simulink model "cpusimuilater"  (R2020b)
settings: Solver=VariableStepAuto  StartTime=0.0  StopTime=inf  RelTol=1e-3
libraries: dspsigops x7
settings Model: Creator=nahomnegash  LastModifiedBy=nahomnegash

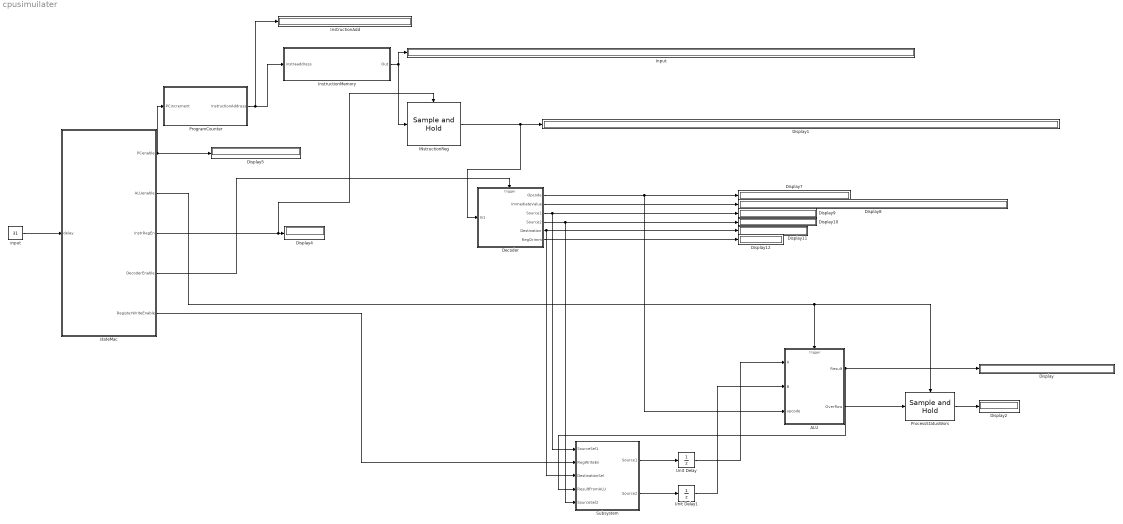
== system cpusimuilater ==
  ALU : Subsystem
  Decoder : Subsystem
  Display{,1..2,4..5,7..12} (11 alike) : Display
  INstructionReg : dspsigops/Sample and Hold  trig=Rising edge  initCond=0  latchinput=off
  Input : Display
  InstructionAdd : Display
  InstructionMemory : Subsystem
  ProcessStatusWors : dspsigops/Sample and Hold  trig=Rising edge  initCond=0  latchinput=off
  ProgramCounter : Subsystem
  Subsystem : Subsystem
  Unit Delay : UnitDelay  SampleTime=-1  HasFrameUpgradeWarning=on
  Unit Delay1 : UnitDelay  SampleTime=-1  HasFrameUpgradeWarning=on
  input : Constant  Value=31
  stateMac : Stateflow chart  TreatAsAtomicUnit=on
      settings: PortSchema="{\"entries\":[{\"content\":{\"sides\":[{\"content\":{\"connectorIds\":[\"In1\"]},\"type\":\"ConnectorPlacement.EquallySpacedRectSide\",\"uuid\":\"cf5c0f17-ae05-41cb-bb8a-264dbf8341ef\"},{\"content\":{\"connectorIds\":[\"Out1\",\"Out4\",\"Out2\",\"Out3\",\"Out5\"],\"side\":\"RIGHT\"},\"type\":\"ConnectorPlacement.EquallySpacedRectSide\",\"uuid\":\"f93a21af-1352-4f9d-82fe-283fa2f49b54\"},{\"content\":{\"connectorIds\":[],\"side\":\"TOP\"},\"type\":\"ConnectorPlacement.EquallySpacedRectSide\",\"uuid\":\"563b2710-7bdc-4fe1-815e-effac7f81df2\"}]},\"type\":\"ConnectorPlacement.EquallySpacedConnector\",\"uuid\":\"4ff43e67-6467-4fb9-af4e-bcbc08840be8\"}],\"packageUris\":[\"http://schema.mathworks.com/mf0/Connector/19700101\"],\"version\":\"1.0\"}"
  wires:
  ALU/1(Result) -> Subsystem/4(ResultFromALU), Display/1
  input/1 -> stateMac/1(delay)
  stateMac/2(InstrRegEn) -> INstructionReg/Trigger, Display4/1
  stateMac/3(DecoderEnable) -> Decoder/Trigger
  stateMac/4(ALUenable) -> ProcessStatusWors/Trigger, ALU/Trigger
  Decoder/2(ImmediateValue) -> Display8/1
  Decoder/3(Source1) -> Subsystem/1(SourceSel1), Display9/1
  Decoder/4(Source2) -> Subsystem/5(SourceSel2), Display10/1
  Decoder/5(Destination) -> Subsystem/3(DestinationSel), Display11/1
  Decoder/6(RegOrimm) -> Display12/1
  Decoder/1(Opcode) -> Display7/1, ALU/3(opcode)
  ALU/2(Overflow) -> ProcessStatusWors/1
  ProcessStatusWors/1 -> Display2/1
  InstructionMemory/1(Out) -> INstructionReg/1, Input/1
  stateMac/5(RegisterWriteEnable) -> Subsystem/2(RegWriteEn)
  INstructionReg/1 -> Decoder/1(In1), Display1/1
  stateMac/1(PCenable) -> Display5/1, ProgramCounter/1(PCincrement)
  ProgramCounter/1(InstructionAddress) -> InstructionMemory/1(instraaddress), InstructionAdd/1
  Subsystem/1(Source1) -> Unit Delay/1
  Unit Delay/1 -> ALU/1(A)
  Unit Delay1/1 -> ALU/2(B)
  Subsystem/2(Source2) -> Unit Delay1/1

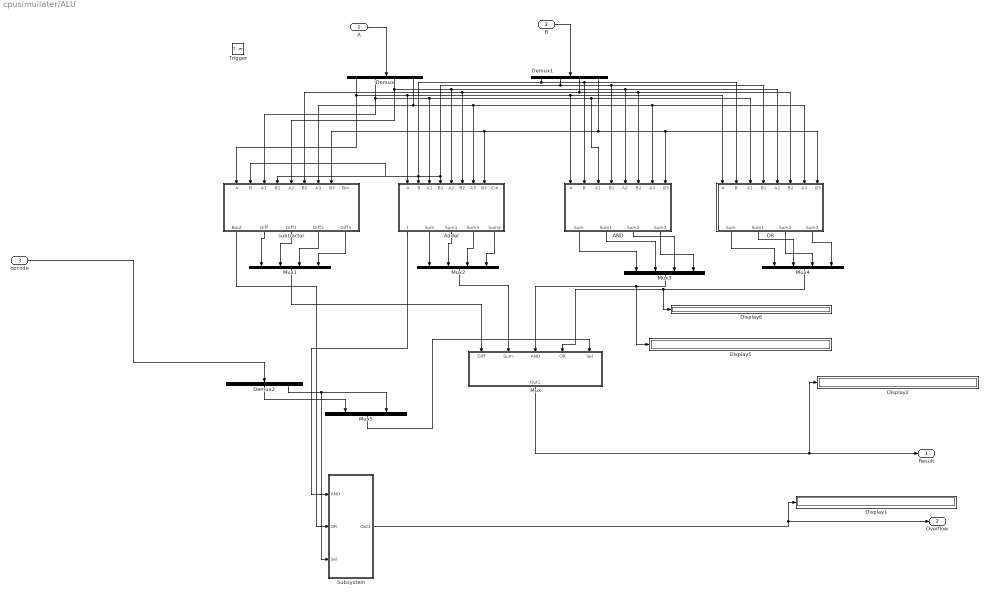
== system cpusimuilater/ALU ==
  A : Inport
  B : Inport  Port=2
  opcode : Inport  Port=3
  Trigger : TriggerPort  VariantControl=Variant  PortDimensions=1
  AND : Subsystem
  Adder : Subsystem
  Demux : Demux
  Demux1 : Demux
  Demux2 : Demux  Outputs=3
  Display{1..2,5..6} (4 alike) : Display
  Mux : Subsystem
  Mux{1..4} (4 alike) : Mux
  Mux5 : Mux  Inputs=2
  OR : Subsystem
  Subsystem : Subsystem
  subtractor : Subsystem
  Result : Outport
  Overflow : Outport  Port=2
  wires:
  A/1 -> Demux/1
  Mux2/1 -> Mux/2(Sum)
  AND/2(Sum1) -> Mux3/2
  Mux/1(Out1) -> Display2/1, Result/1
  Adder/1(CarryOut) -> Subsystem/1(AND)
  opcode/1 -> Demux2/1
  OR/4(Sum3) -> Mux4/4
  B/1 -> Demux1/1
  subtractor/1(Bout) -> Subsystem/2(OR)
  OR/1(Sum) -> Mux4/1
  Mux5/1 -> Mux/5(Sel)
  subtractor/5(Diff3) -> Mux1/4
  Mux4/1 -> Display6/1, Mux/4(OR)
  Mux3/1 -> Display5/1, Mux/3(AND)
  Adder/3(Sum1) -> Mux2/2
  Demux2/2 -> Mux5/1
  Adder/2(Sum) -> Mux2/1
  subtractor/2(Diff) -> Mux1/1
  Demux2/3 -> Subsystem/3(Sel), Mux5/2
  AND/1(Sum) -> Mux3/1
  Adder/5(Sum2) -> Mux2/4
  Mux1/1 -> Mux/1(Diff)
  OR/2(Sum1) -> Mux4/2
  AND/4(Sum3) -> Mux3/4
  subtractor/3(Diff1) -> Mux1/2
  OR/3(Sum2) -> Mux4/3
  subtractor/4(Diff2) -> Mux1/3
  AND/3(Sum2) -> Mux3/3
  Subsystem/1(Out1) -> Display1/1, Overflow/1
  Adder/4(Sum3) -> Mux2/3
  Demux1/4 -> subtractor/8(B3), Adder/8(B3), OR/8(B3), AND/8(B3)
  Demux/4 -> subtractor/7(A3), Adder/7(A3), AND/7(A3), OR/7(A3)
  Demux1/3 -> subtractor/6(B2), Adder/6(B2), AND/6(B2), OR/6(B2)
  Demux1/2 -> subtractor/4(B1), Adder/4(B1), AND/4(B1), OR/4(B1)
  Demux1/1 -> subtractor/2(B), Adder/2(B), AND/2(B), OR/2(B)
  Demux/3 -> subtractor/5(A2), Adder/5(A2), AND/5(A2), OR/5(A2)
  Demux/2 -> subtractor/3(A1), Adder/3(A1), OR/3(A1), AND/3(A1)
  Demux/1 -> subtractor/1(A), Adder/1(A), AND/1(A), OR/1(A)

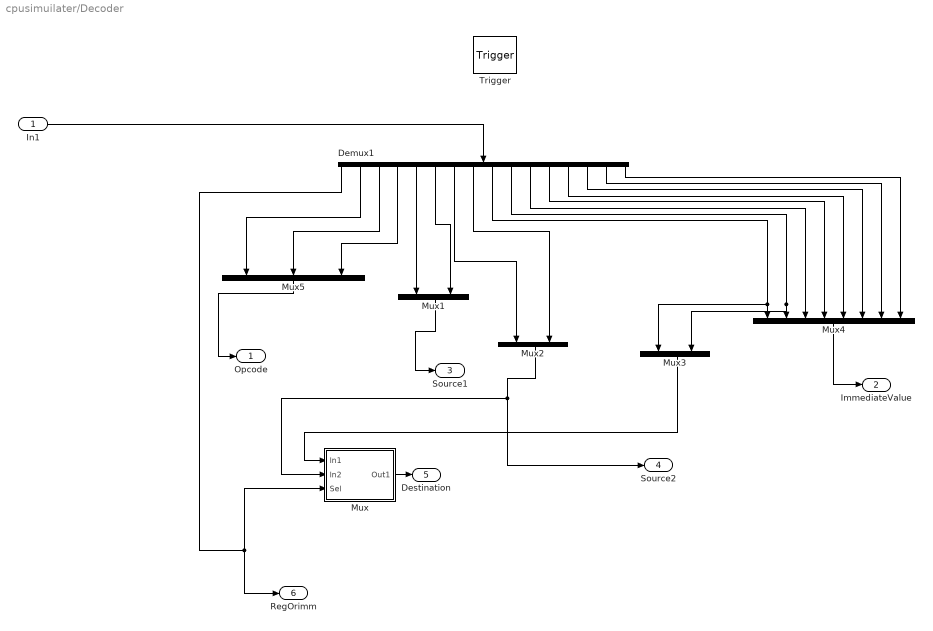
== system cpusimuilater/Decoder ==
  In1 : Inport
  Trigger : TriggerPort  VariantControl=Variant  PortDimensions=1
  Demux1 : Demux  Outputs=16
  Mux : Subsystem
  Mux1 : Mux  Inputs=2
  Mux2 : Mux  Inputs=2
  Mux3 : Mux  Inputs=2
  Mux4 : Mux  Inputs=8
  Mux5 : Mux  Inputs=3
  Opcode : Outport
  ImmediateValue : Outport  Port=2
  Source1 : Outport  Port=3
  Source2 : Outport  Port=4
  Destination : Outport  Port=5
  RegOrimm : Outport  Port=6
  wires:
  Demux1/13 -> Mux4/5
  Demux1/16 -> Mux4/8
  Mux3/1 -> Mux/1(ln1)
  Mux1/1 -> Source1/1
  Demux1/14 -> Mux4/6
  Demux1/6 -> Mux1/2
  Demux1/11 -> Mux4/3
  Demux1/7 -> Mux2/1
  In1/1 -> Demux1/1
  Demux1/9 -> Mux3/1, Mux4/1
  Demux1/4 -> Mux5/3
  Demux1/8 -> Mux2/2
  Demux1/3 -> Mux5/2
  Mux5/1 -> Opcode/1
  Demux1/10 -> Mux3/2, Mux4/2
  Mux2/1 -> Source2/1, Mux/2(ln2)
  Demux1/5 -> Mux1/1
  Mux/1(Out1) -> Destination/1
  Demux1/15 -> Mux4/7
  Demux1/1 -> RegOrimm/1, Mux/3(Sel)
  Mux4/1 -> ImmediateValue/1
  Demux1/12 -> Mux4/4
  Demux1/2 -> Mux5/1

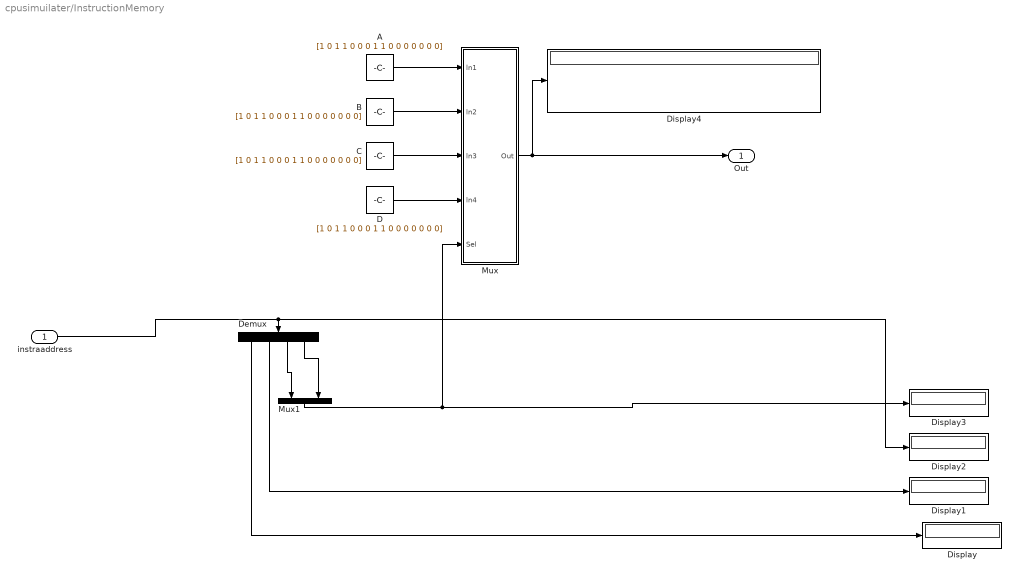
== system cpusimuilater/InstructionMemory ==
  instraaddress : Inport
  A : Constant  Value=[1 0 1 1 0 0 0 1 1 0 0 0 0 0 0 0]
  B : Constant  Value=[1 0 1 1 0 0 0 1 1 0 0 0 0 0 0 0]
  C : Constant  Value=[1 0 1 1 0 0 0 1 1 0 0 0 0 0 0 0]
  D : Constant  Value=[1 0 1 1 0 0 0 1 1 0 0 0 0 0 0 0]
  Demux : Demux
  Display{,1..4} (5 alike) : Display
  Mux : Subsystem
  Mux1 : Mux  Inputs=2
  Out : Outport
  wires:
  instraaddress/1 -> Display2/1, Demux/1
  Mux/1(Out) -> Out/1, Display4/1
  Demux/4 -> Mux1/2
  Demux/3 -> Mux1/1
  Mux1/1 -> Display3/1, Mux/5(Sel)
  A/1 -> Mux/1(ln1)
  B/1 -> Mux/2(ln2)
  C/1 -> Mux/3(ln3)
  D/1 -> Mux/4(ln4)
  Demux/1 -> Display/1
  Demux/2 -> Display1/1

== system cpusimuilater/ProgramCounter ==
  PCincrement : Inport
  Adder1 : Subsystem
  Constant : Constant
  Constant1 : Constant
  Demux : Demux
  Display : Display
  Display1 : Display
  Mux2 : Mux
  Sample and Hold : dspsigops/Sample and Hold  trig=Rising edge  initCond=0  latchinput=off
  Unit Delay : UnitDelay  SampleTime=-1  HasFrameUpgradeWarning=on
  InstructionAddress : Outport
  wires:
  Mux2/1 -> InstructionAddress/1, Display1/1, Unit Delay/1
  Adder1/1(CarryOut) -> Display/1
  Adder1/3(Sum1) -> Mux2/2
  Unit Delay/1 -> Sample and Hold/1
  Sample and Hold/1 -> Demux/1
  Adder1/2(Sum) -> Mux2/1
  Constant1/1 -> Adder1/9(C), Adder1/6(B2), Adder1/4(B1), Adder1/2(B)
  Adder1/5(Sum3) -> Mux2/4
  Demux/2 -> Adder1/3(A1)
  Adder1/4(Sum2) -> Mux2/3
  Constant/1 -> Adder1/8(B3)
  Demux/1 -> Adder1/1(A)
  Demux/3 -> Adder1/5(A2)
  Demux/4 -> Adder1/7(A3)
  PCincrement/1 -> Sample and Hold/Trigger

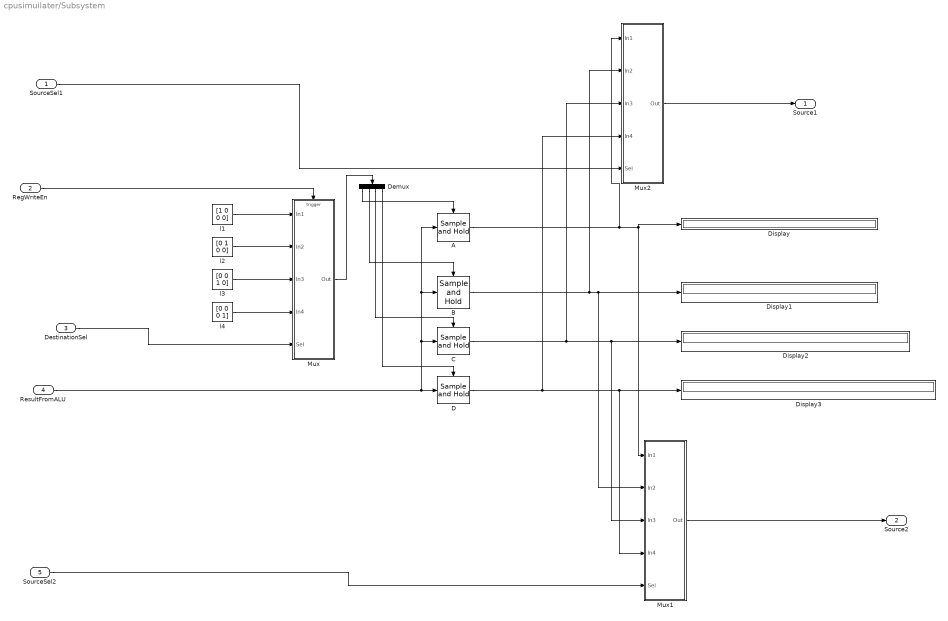
== system cpusimuilater/Subsystem ==
  SourceSel1 : Inport
  RegWriteEn : Inport  Port=2
  DestinationSel : Inport  Port=3
  ResultFromALU : Inport  Port=4
  SourceSel2 : Inport  Port=5
  A : dspsigops/Sample and Hold  trig=Rising edge  initCond=[1 0 0 0]  latchinput=off
  B : dspsigops/Sample and Hold  trig=Rising edge  initCond=[0 1 0 0]  latchinput=off
  C : dspsigops/Sample and Hold  trig=Rising edge  initCond=[0 0 1 0]  latchinput=off
  D : dspsigops/Sample and Hold  trig=Rising edge  initCond=[0 0 0 0]  latchinput=off
  Demux : Demux
  Display{,1..3} (4 alike) : Display
  Mux : Subsystem
  Mux1 : Subsystem
  Mux2 : Subsystem
  l1 : Constant  Value=[1 0 0 0]
  l2 : Constant  Value=[0 1 0 0]
  l3 : Constant  Value=[0 0 1 0]
  l4 : Constant  Value=[0 0 0 1]
  Source1 : Outport
  Source2 : Outport  Port=2
  wires:
  SourceSel1/1 -> Mux2/5(Sel)
  DestinationSel/1 -> Mux/5(Sel)
  Demux/4 -> D/Trigger
  l3/1 -> Mux/3(ln3)
  l2/1 -> Mux/2(ln2)
  Demux/3 -> C/Trigger
  Mux/1(Out) -> Demux/1
  l1/1 -> Mux/1(ln1)
  SourceSel2/1 -> Mux1/5(Sel)
  Mux1/1(Out) -> Source2/1
  l4/1 -> Mux/4(ln4)
  Demux/2 -> B/Trigger
  B/1 -> Display1/1, Mux1/2(ln2), Mux2/2(ln2)
  RegWriteEn/1 -> Mux/Trigger
  Mux2/1(Out) -> Source1/1
  D/1 -> Display3/1, Mux1/4(ln4), Mux2/4(ln4)
  A/1 -> Mux2/1(ln1), Mux1/1(ln1), Display/1
  Demux/1 -> A/Trigger
  ResultFromALU/1 -> A/1, B/1, C/1, D/1
  C/1 -> Display2/1, Mux1/3(ln3), Mux2/3(ln3)

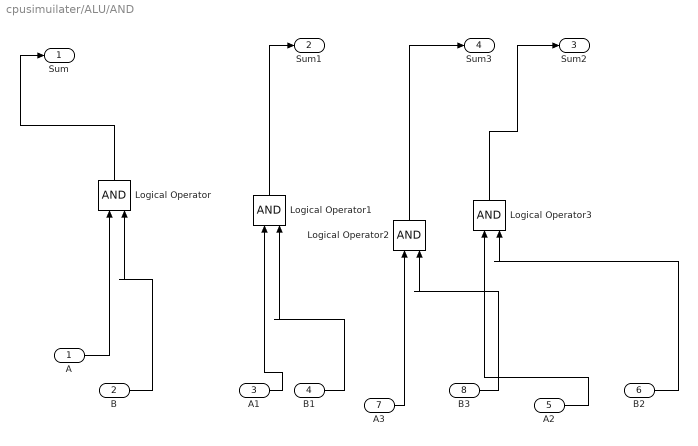
== system cpusimuilater/ALU/AND ==
  A : Inport
  B : Inport  Port=2
  A1 : Inport  Port=3
  B1 : Inport  Port=4
  A2 : Inport  Port=5
  B2 : Inport  Port=6
  A3 : Inport  Port=7
  B3 : Inport  Port=8
  Logical Operator{,1..3} (4 alike) : Logic  IconShape=distinctive  AllPortsSameDT=off  OutDataTypeStr=boolean
  Sum : Outport
  Sum1 : Outport  Port=2
  Sum2 : Outport  Port=3
  Sum3 : Outport  Port=4
  wires:
  A2/1 -> Logical Operator3/1
  Logical Operator2/1 -> Sum3/1
  B/1 -> Logical Operator/2
  B1/1 -> Logical Operator1/2
  A1/1 -> Logical Operator1/1
  B2/1 -> Logical Operator3/2
  A3/1 -> Logical Operator2/1
  Logical Operator3/1 -> Sum2/1
  B3/1 -> Logical Operator2/2
  Logical Operator1/1 -> Sum1/1
  Logical Operator/1 -> Sum/1
  A/1 -> Logical Operator/1

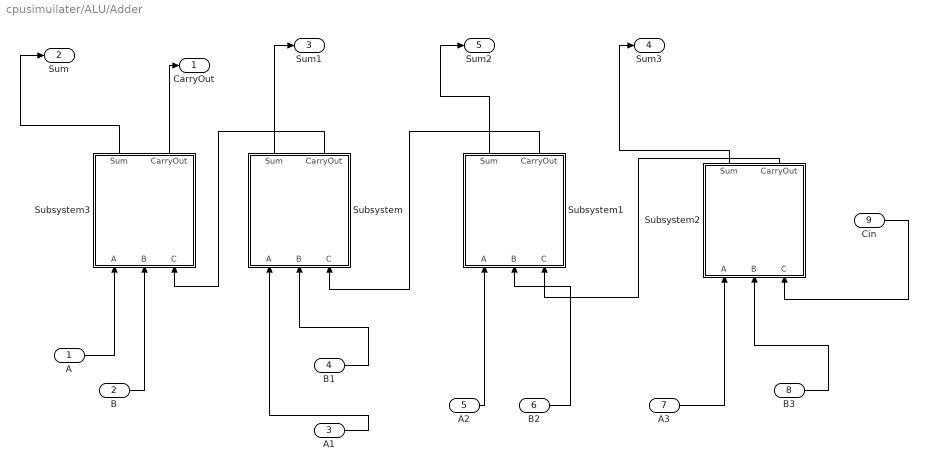
== system cpusimuilater/ALU/Adder ==
  A : Inport
  B : Inport  Port=2
  A1 : Inport  Port=3
  B1 : Inport  Port=4
  A2 : Inport  Port=5
  B2 : Inport  Port=6
  A3 : Inport  Port=7
  B3 : Inport  Port=8
  Cin : Inport  Port=9
  Subsystem : Subsystem
  Subsystem1 : Subsystem
  Subsystem2 : Subsystem
  Subsystem3 : Subsystem
  CarryOut : Outport
  Sum : Outport  Port=2
  Sum1 : Outport  Port=3
  Sum3 : Outport  Port=4
  Sum2 : Outport  Port=5
  wires:
  A2/1 -> Subsystem1/1(A)
  B1/1 -> Subsystem/2(B)
  Subsystem1/1(Sum) -> Sum2/1
  Subsystem/1(Sum) -> Sum1/1
  Subsystem2/1(Sum) -> Sum3/1
  B2/1 -> Subsystem1/2(B)
  Subsystem3/1(Sum) -> Sum/1
  A1/1 -> Subsystem/1(A)
  B3/1 -> Subsystem2/2(B)
  A3/1 -> Subsystem2/1(A)
  A/1 -> Subsystem3/1(A)
  B/1 -> Subsystem3/2(B)
  Subsystem2/2(CarryOut) -> Subsystem1/3(C)
  Subsystem/2(CarryOut) -> Subsystem3/3(C)
  Subsystem1/2(CarryOut) -> Subsystem/3(C)
  Subsystem3/2(CarryOut) -> CarryOut/1
  Cin/1 -> Subsystem2/3(C)

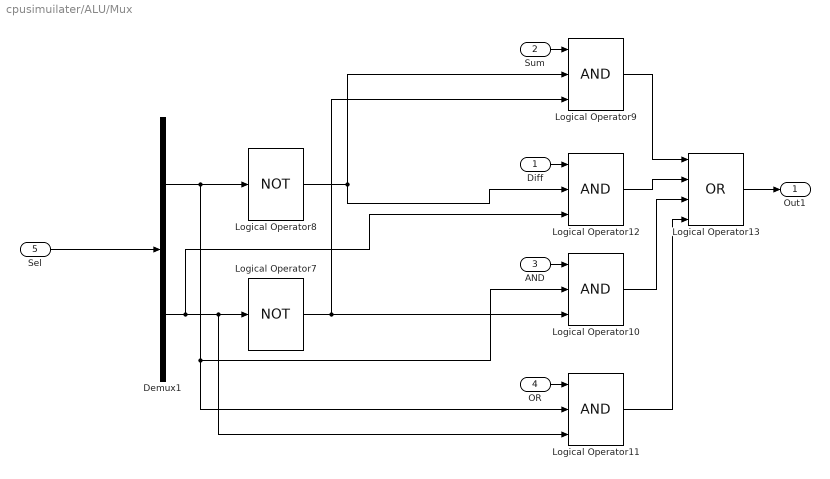
== system cpusimuilater/ALU/Mux ==
  Diff : Inport
  Sum : Inport  Port=2
  AND : Inport  Port=3
  OR : Inport  Port=4
  Sel : Inport  Port=5
  Demux1 : Demux  Outputs=2
  Logical Operator{9..12} (4 alike) : Logic  Inputs=3  IconShape=distinctive  AllPortsSameDT=off  OutDataTypeStr=boolean
  Logical Operator13 : Logic  Operator=OR  Inputs=4  IconShape=distinctive  AllPortsSameDT=off  OutDataTypeStr=boolean
  Logical Operator7 : Logic  Operator=NOT  Inputs=1  IconShape=distinctive  AllPortsSameDT=off  OutDataTypeStr=boolean
  Logical Operator8 : Logic  Operator=NOT  Inputs=1  IconShape=distinctive  AllPortsSameDT=off  OutDataTypeStr=boolean
  Out1 : Outport
  wires:
  AND/1 -> Logical Operator10/1
  OR/1 -> Logical Operator11/1
  Diff/1 -> Logical Operator12/1
  Logical Operator11/1 -> Logical Operator13/4
  Logical Operator10/1 -> Logical Operator13/3
  Logical Operator8/1 -> Logical Operator12/2, Logical Operator9/2
  Logical Operator9/1 -> Logical Operator13/1
  Logical Operator13/1 -> Out1/1
  Demux1/1 -> Logical Operator8/1, Logical Operator10/2, Logical Operator11/2
  Sum/1 -> Logical Operator9/1
  Logical Operator7/1 -> Logical Operator9/3, Logical Operator10/3
  Logical Operator12/1 -> Logical Operator13/2
  Demux1/2 -> Logical Operator12/3, Logical Operator11/3, Logical Operator7/1
  Sel/1 -> Demux1/1

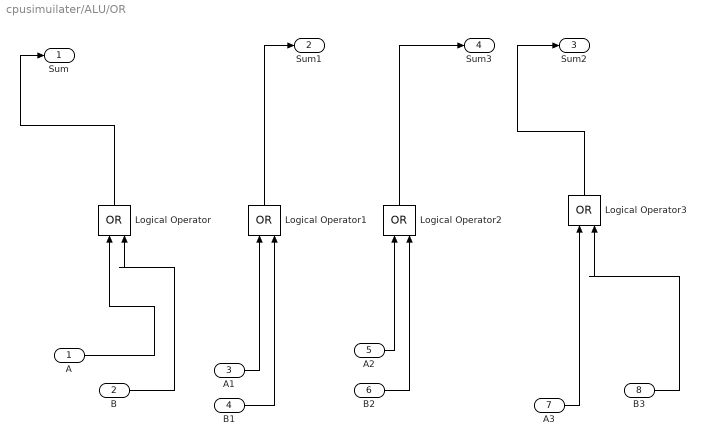
== system cpusimuilater/ALU/OR ==
  A : Inport
  B : Inport  Port=2
  A1 : Inport  Port=3
  B1 : Inport  Port=4
  A2 : Inport  Port=5
  B2 : Inport  Port=6
  A3 : Inport  Port=7
  B3 : Inport  Port=8
  Logical Operator{,1..3} (4 alike) : Logic  Operator=OR  IconShape=distinctive  AllPortsSameDT=off  OutDataTypeStr=boolean
  Sum : Outport
  Sum1 : Outport  Port=2
  Sum2 : Outport  Port=3
  Sum3 : Outport  Port=4
  wires:
  A3/1 -> Logical Operator3/1
  Logical Operator2/1 -> Sum3/1
  B/1 -> Logical Operator/2
  B1/1 -> Logical Operator1/2
  A1/1 -> Logical Operator1/1
  B3/1 -> Logical Operator3/2
  A2/1 -> Logical Operator2/1
  Logical Operator3/1 -> Sum2/1
  B2/1 -> Logical Operator2/2
  Logical Operator1/1 -> Sum1/1
  Logical Operator/1 -> Sum/1
  A/1 -> Logical Operator/1

== system cpusimuilater/ALU/Subsystem ==
  AND : Inport
  OR : Inport  Port=2
  Sel : Inport  Port=3
  Logical Operator10 : Logic  IconShape=distinctive  AllPortsSameDT=off  OutDataTypeStr=boolean
  Logical Operator11 : Logic  IconShape=distinctive  AllPortsSameDT=off  OutDataTypeStr=boolean
  Logical Operator13 : Logic  Operator=OR  IconShape=distinctive  AllPortsSameDT=off  OutDataTypeStr=boolean
  Logical Operator7 : Logic  Operator=NOT  Inputs=1  IconShape=distinctive  AllPortsSameDT=off  OutDataTypeStr=boolean
  Out1 : Outport
  wires:
  Logical Operator7/1 -> Logical Operator10/2
  Sel/1 -> Logical Operator11/2, Logical Operator7/1
  AND/1 -> Logical Operator10/1
  Logical Operator13/1 -> Out1/1
  OR/1 -> Logical Operator11/1
  Logical Operator11/1 -> Logical Operator13/2
  Logical Operator10/1 -> Logical Operator13/1

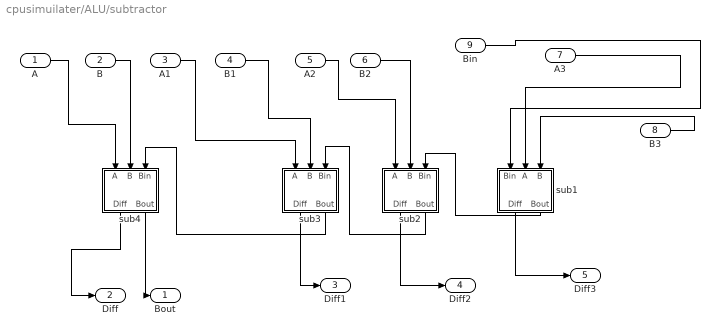
== system cpusimuilater/ALU/subtractor ==
  A : Inport
  B : Inport  Port=2
  A1 : Inport  Port=3
  B1 : Inport  Port=4
  A2 : Inport  Port=5
  B2 : Inport  Port=6
  A3 : Inport  Port=7
  B3 : Inport  Port=8
  Bin : Inport  Port=9
  sub1 : Subsystem
  sub2 : Subsystem
  sub3 : Subsystem
  sub4 : Subsystem
  Bout : Outport
  Diff : Outport  Port=2
  Diff1 : Outport  Port=3
  Diff2 : Outport  Port=4
  Diff3 : Outport  Port=5
  wires:
  B1/1 -> sub3/2(B)
  sub4/1(Diff) -> Diff/1
  A3/1 -> sub1/2(A)
  sub3/1(Diff) -> Diff1/1
  A1/1 -> sub3/1(A)
  sub1/2(Bout) -> sub2/3(Bin)
  A/1 -> sub4/1(A)
  B/1 -> sub4/2(B)
  sub2/2(Bout) -> sub3/3(Bin)
  A2/1 -> sub2/1(A)
  Bin/1 -> sub1/1(Bin)
  sub1/1(Diff) -> Diff3/1
  sub3/2(Bout) -> sub4/3(Bin)
  sub2/1(Diff) -> Diff2/1
  B2/1 -> sub2/2(B)
  sub4/2(Bout) -> Bout/1
  B3/1 -> sub1/3(B)

== system cpusimuilater/Decoder/Mux ==
  ln1 : Inport
  ln2 : Inport  Port=2
  Sel : Inport  Port=3
  Logical Operator10 : Logic  IconShape=distinctive  AllPortsSameDT=off  OutDataTypeStr=boolean
  Logical Operator11 : Logic  IconShape=distinctive  AllPortsSameDT=off  OutDataTypeStr=boolean
  Logical Operator13 : Logic  Operator=OR  IconShape=distinctive  AllPortsSameDT=off  OutDataTypeStr=boolean
  Logical Operator7 : Logic  Operator=NOT  Inputs=1  IconShape=distinctive  AllPortsSameDT=off  OutDataTypeStr=boolean
  Out1 : Outport
  wires:
  Logical Operator10/1 -> Logical Operator13/1
  Logical Operator11/1 -> Logical Operator13/2
  ln2/1 -> Logical Operator11/1
  Logical Operator13/1 -> Out1/1
  ln1/1 -> Logical Operator10/1
  Sel/1 -> Logical Operator7/1, Logical Operator11/2
  Logical Operator7/1 -> Logical Operator10/2

== system cpusimuilater/InstructionMemory/Mux ==
  ln1 : Inport
  ln2 : Inport  Port=2
  ln3 : Inport  Port=3
  ln4 : Inport  Port=4
  Sel : Inport  Port=5
  Demux1 : Demux  Outputs=2
  Logical Operator{9..12} (4 alike) : Logic  Inputs=3  IconShape=distinctive  AllPortsSameDT=off  OutDataTypeStr=boolean
  Logical Operator13 : Logic  Operator=OR  Inputs=4  IconShape=distinctive  AllPortsSameDT=off  OutDataTypeStr=boolean
  Logical Operator7 : Logic  Operator=NOT  Inputs=1  IconShape=distinctive  AllPortsSameDT=off  OutDataTypeStr=boolean
  Logical Operator8 : Logic  Operator=NOT  Inputs=1  IconShape=distinctive  AllPortsSameDT=off  OutDataTypeStr=boolean
  Out : Outport
  wires:
  ln3/1 -> Logical Operator10/1
  ln4/1 -> Logical Operator11/1
  ln2/1 -> Logical Operator12/1
  Logical Operator11/1 -> Logical Operator13/4
  Logical Operator10/1 -> Logical Operator13/3
  Logical Operator8/1 -> Logical Operator12/2, Logical Operator9/2
  Logical Operator9/1 -> Logical Operator13/1
  Logical Operator13/1 -> Out/1
  Demux1/1 -> Logical Operator8/1, Logical Operator10/2, Logical Operator11/2
  ln1/1 -> Logical Operator9/1
  Logical Operator7/1 -> Logical Operator9/3, Logical Operator10/3
  Logical Operator12/1 -> Logical Operator13/2
  Demux1/2 -> Logical Operator12/3, Logical Operator11/3, Logical Operator7/1
  Sel/1 -> Demux1/1

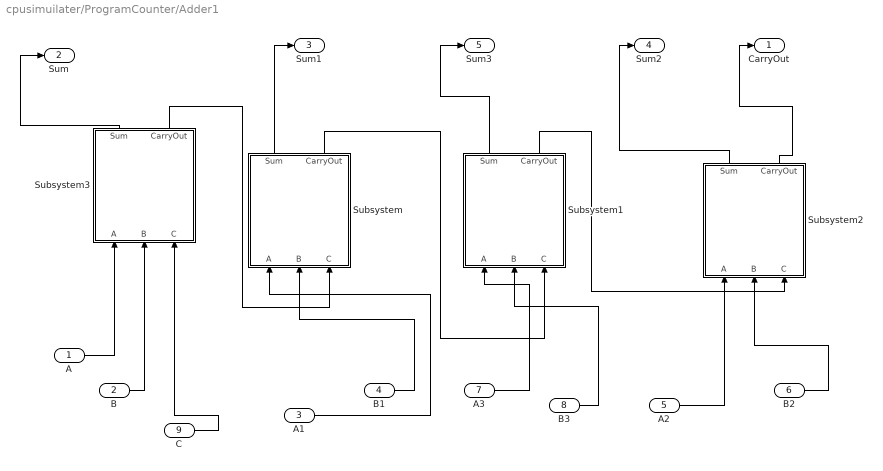
== system cpusimuilater/ProgramCounter/Adder1 ==
  A : Inport
  B : Inport  Port=2
  A1 : Inport  Port=3
  B1 : Inport  Port=4
  A2 : Inport  Port=5
  B2 : Inport  Port=6
  A3 : Inport  Port=7
  B3 : Inport  Port=8
  C : Inport  Port=9
  Subsystem : Subsystem
  Subsystem1 : Subsystem
  Subsystem2 : Subsystem
  Subsystem3 : Subsystem
  CarryOut : Outport
  Sum : Outport  Port=2
  Sum1 : Outport  Port=3
  Sum2 : Outport  Port=4
  Sum3 : Outport  Port=5
  wires:
  A3/1 -> Subsystem1/1(A)
  B1/1 -> Subsystem/2(B)
  Subsystem1/1(Sum) -> Sum3/1
  A/1 -> Subsystem3/1(A)
  Subsystem/1(Sum) -> Sum1/1
  Subsystem3/2(CarryOut) -> Subsystem/3(C)
  Subsystem2/1(Sum) -> Sum2/1
  Subsystem/2(CarryOut) -> Subsystem1/3(C)
  B3/1 -> Subsystem1/2(B)
  Subsystem3/1(Sum) -> Sum/1
  B/1 -> Subsystem3/2(B)
  C/1 -> Subsystem3/3(C)
  Subsystem2/2(CarryOut) -> CarryOut/1
  A1/1 -> Subsystem/1(A)
  Subsystem1/2(CarryOut) -> Subsystem2/3(C)
  B2/1 -> Subsystem2/2(B)
  A2/1 -> Subsystem2/1(A)

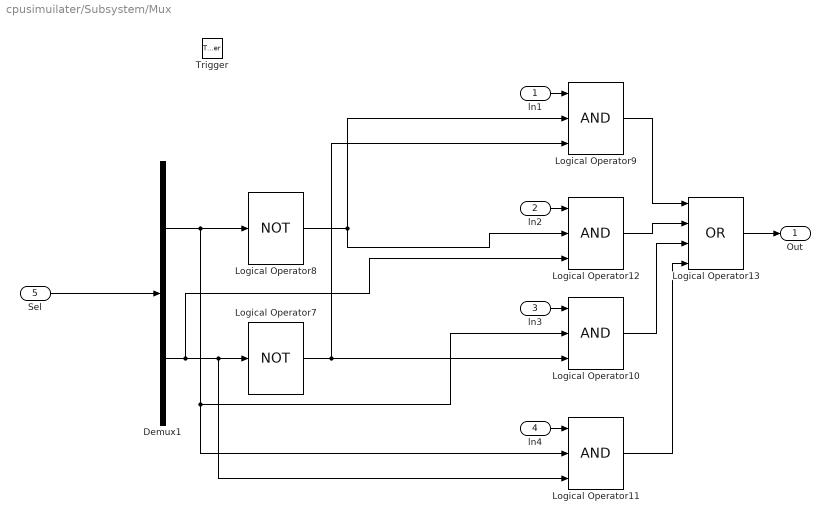
== system cpusimuilater/Subsystem/Mux ==
  ln1 : Inport
  ln2 : Inport  Port=2
  ln3 : Inport  Port=3
  ln4 : Inport  Port=4
  Sel : Inport  Port=5
  Trigger : TriggerPort  VariantControl=Variant  PortDimensions=1
  Demux1 : Demux  Outputs=2
  Logical Operator{9..12} (4 alike) : Logic  Inputs=3  IconShape=distinctive  AllPortsSameDT=off  OutDataTypeStr=boolean
  Logical Operator13 : Logic  Operator=OR  Inputs=4  IconShape=distinctive  AllPortsSameDT=off  OutDataTypeStr=boolean
  Logical Operator7 : Logic  Operator=NOT  Inputs=1  IconShape=distinctive  AllPortsSameDT=off  OutDataTypeStr=boolean
  Logical Operator8 : Logic  Operator=NOT  Inputs=1  IconShape=distinctive  AllPortsSameDT=off  OutDataTypeStr=boolean
  Out : Outport
  wires:
  ln3/1 -> Logical Operator10/1
  ln4/1 -> Logical Operator11/1
  ln2/1 -> Logical Operator12/1
  Logical Operator11/1 -> Logical Operator13/4
  Logical Operator10/1 -> Logical Operator13/3
  Logical Operator8/1 -> Logical Operator12/2, Logical Operator9/2
  Logical Operator9/1 -> Logical Operator13/1
  Logical Operator13/1 -> Out/1
  Demux1/1 -> Logical Operator8/1, Logical Operator10/2, Logical Operator11/2
  ln1/1 -> Logical Operator9/1
  Logical Operator7/1 -> Logical Operator9/3, Logical Operator10/3
  Logical Operator12/1 -> Logical Operator13/2
  Demux1/2 -> Logical Operator12/3, Logical Operator11/3, Logical Operator7/1
  Sel/1 -> Demux1/1

== system cpusimuilater/Subsystem/Mux1 ==
  ln1 : Inport
  ln2 : Inport  Port=2
  ln3 : Inport  Port=3
  ln4 : Inport  Port=4
  Sel : Inport  Port=5
  Demux1 : Demux  Outputs=2
  Logical Operator{9..12} (4 alike) : Logic  Inputs=3  IconShape=distinctive  AllPortsSameDT=off  OutDataTypeStr=boolean
  Logical Operator13 : Logic  Operator=OR  Inputs=4  IconShape=distinctive  AllPortsSameDT=off  OutDataTypeStr=boolean
  Logical Operator7 : Logic  Operator=NOT  Inputs=1  IconShape=distinctive  AllPortsSameDT=off  OutDataTypeStr=boolean
  Logical Operator8 : Logic  Operator=NOT  Inputs=1  IconShape=distinctive  AllPortsSameDT=off  OutDataTypeStr=boolean
  Out : Outport
  wires:
  Sel/1 -> Demux1/1
  Demux1/2 -> Logical Operator7/1, Logical Operator11/3, Logical Operator12/3
  Logical Operator12/1 -> Logical Operator13/2
  Logical Operator7/1 -> Logical Operator10/3, Logical Operator9/3
  ln1/1 -> Logical Operator9/1
  Demux1/1 -> Logical Operator11/2, Logical Operator10/2, Logical Operator8/1
  Logical Operator13/1 -> Out/1
  Logical Operator9/1 -> Logical Operator13/1
  Logical Operator8/1 -> Logical Operator9/2, Logical Operator12/2
  Logical Operator10/1 -> Logical Operator13/3
  Logical Operator11/1 -> Logical Operator13/4
  ln2/1 -> Logical Operator12/1
  ln4/1 -> Logical Operator11/1
  ln3/1 -> Logical Operator10/1

== system cpusimuilater/Subsystem/Mux2 ==
  ln1 : Inport
  ln2 : Inport  Port=2
  ln3 : Inport  Port=3
  ln4 : Inport  Port=4
  Sel : Inport  Port=5
  Demux1 : Demux  Outputs=2
  Logical Operator{9..12} (4 alike) : Logic  Inputs=3  IconShape=distinctive  AllPortsSameDT=off  OutDataTypeStr=boolean
  Logical Operator13 : Logic  Operator=OR  Inputs=4  IconShape=distinctive  AllPortsSameDT=off  OutDataTypeStr=boolean
  Logical Operator7 : Logic  Operator=NOT  Inputs=1  IconShape=distinctive  AllPortsSameDT=off  OutDataTypeStr=boolean
  Logical Operator8 : Logic  Operator=NOT  Inputs=1  IconShape=distinctive  AllPortsSameDT=off  OutDataTypeStr=boolean
  Out : Outport
  wires:
  ln3/1 -> Logical Operator10/1
  ln4/1 -> Logical Operator11/1
  ln2/1 -> Logical Operator12/1
  Logical Operator11/1 -> Logical Operator13/4
  Logical Operator10/1 -> Logical Operator13/3
  Logical Operator8/1 -> Logical Operator12/2, Logical Operator9/2
  Logical Operator9/1 -> Logical Operator13/1
  Logical Operator13/1 -> Out/1
  Demux1/1 -> Logical Operator8/1, Logical Operator10/2, Logical Operator11/2
  ln1/1 -> Logical Operator9/1
  Logical Operator7/1 -> Logical Operator9/3, Logical Operator10/3
  Logical Operator12/1 -> Logical Operator13/2
  Demux1/2 -> Logical Operator12/3, Logical Operator11/3, Logical Operator7/1
  Sel/1 -> Demux1/1

== system cpusimuilater/ALU/Adder/Subsystem ==
  A : Inport
  B : Inport  Port=2
  C : Inport  Port=3
  Logical Operator : Logic  Operator=XOR  IconShape=distinctive  AllPortsSameDT=off  OutDataTypeStr=boolean
  Logical Operator1 : Logic  IconShape=distinctive  AllPortsSameDT=off  OutDataTypeStr=boolean
  Logical Operator3 : Logic  Operator=OR  IconShape=distinctive  AllPortsSameDT=off  OutDataTypeStr=boolean
  Logical Operator4 : Logic  Operator=XOR  IconShape=distinctive  AllPortsSameDT=off  OutDataTypeStr=boolean
  Logical Operator5 : Logic  IconShape=distinctive  AllPortsSameDT=off  OutDataTypeStr=boolean
  Sum : Outport
  CarryOut : Outport  Port=2
  wires:
  Logical Operator/1 -> Logical Operator4/2, Logical Operator5/1
  Logical Operator5/1 -> Logical Operator3/1
  Logical Operator1/1 -> Logical Operator3/2
  Logical Operator4/1 -> Sum/1
  Logical Operator3/1 -> CarryOut/1
  A/1 -> Logical Operator1/1, Logical Operator/1
  C/1 -> Logical Operator4/1, Logical Operator5/2
  B/1 -> Logical Operator1/2, Logical Operator/2

== system cpusimuilater/ALU/Adder/Subsystem1 ==
  A : Inport
  B : Inport  Port=2
  C : Inport  Port=3
  Logical Operator : Logic  Operator=XOR  IconShape=distinctive  AllPortsSameDT=off  OutDataTypeStr=boolean
  Logical Operator1 : Logic  IconShape=distinctive  AllPortsSameDT=off  OutDataTypeStr=boolean
  Logical Operator3 : Logic  Operator=OR  IconShape=distinctive  AllPortsSameDT=off  OutDataTypeStr=boolean
  Logical Operator4 : Logic  Operator=XOR  IconShape=distinctive  AllPortsSameDT=off  OutDataTypeStr=boolean
  Logical Operator5 : Logic  IconShape=distinctive  AllPortsSameDT=off  OutDataTypeStr=boolean
  Sum : Outport
  CarryOut : Outport  Port=2
  wires:
  Logical Operator/1 -> Logical Operator4/2, Logical Operator5/1
  Logical Operator5/1 -> Logical Operator3/1
  Logical Operator1/1 -> Logical Operator3/2
  Logical Operator4/1 -> Sum/1
  Logical Operator3/1 -> CarryOut/1
  A/1 -> Logical Operator1/1, Logical Operator/1
  C/1 -> Logical Operator4/1, Logical Operator5/2
  B/1 -> Logical Operator1/2, Logical Operator/2

== system cpusimuilater/ALU/Adder/Subsystem2 ==
  A : Inport
  B : Inport  Port=2
  C : Inport  Port=3
  Logical Operator : Logic  Operator=XOR  IconShape=distinctive  AllPortsSameDT=off  OutDataTypeStr=boolean
  Logical Operator1 : Logic  IconShape=distinctive  AllPortsSameDT=off  OutDataTypeStr=boolean
  Logical Operator3 : Logic  Operator=OR  IconShape=distinctive  AllPortsSameDT=off  OutDataTypeStr=boolean
  Logical Operator4 : Logic  Operator=XOR  IconShape=distinctive  AllPortsSameDT=off  OutDataTypeStr=boolean
  Logical Operator5 : Logic  IconShape=distinctive  AllPortsSameDT=off  OutDataTypeStr=boolean
  Sum : Outport
  CarryOut : Outport  Port=2
  wires:
  Logical Operator/1 -> Logical Operator4/2, Logical Operator5/1
  Logical Operator5/1 -> Logical Operator3/1
  Logical Operator1/1 -> Logical Operator3/2
  Logical Operator4/1 -> Sum/1
  Logical Operator3/1 -> CarryOut/1
  A/1 -> Logical Operator1/1, Logical Operator/1
  C/1 -> Logical Operator4/1, Logical Operator5/2
  B/1 -> Logical Operator1/2, Logical Operator/2

== system cpusimuilater/ALU/Adder/Subsystem3 ==
  A : Inport
  B : Inport  Port=2
  C : Inport  Port=3
  Logical Operator : Logic  Operator=XOR  IconShape=distinctive  AllPortsSameDT=off  OutDataTypeStr=boolean
  Logical Operator1 : Logic  IconShape=distinctive  AllPortsSameDT=off  OutDataTypeStr=boolean
  Logical Operator3 : Logic  Operator=OR  IconShape=distinctive  AllPortsSameDT=off  OutDataTypeStr=boolean
  Logical Operator4 : Logic  Operator=XOR  IconShape=distinctive  AllPortsSameDT=off  OutDataTypeStr=boolean
  Logical Operator5 : Logic  IconShape=distinctive  AllPortsSameDT=off  OutDataTypeStr=boolean
  Sum : Outport
  CarryOut : Outport  Port=2
  wires:
  A/1 -> Logical Operator1/1, Logical Operator/1
  Logical Operator5/1 -> Logical Operator3/1
  B/1 -> Logical Operator1/2, Logical Operator/2
  Logical Operator3/1 -> CarryOut/1
  Logical Operator1/1 -> Logical Operator3/2
  Logical Operator4/1 -> Sum/1
  Logical Operator/1 -> Logical Operator4/2, Logical Operator5/1
  C/1 -> Logical Operator4/1, Logical Operator5/2

== system cpusimuilater/ALU/subtractor/sub1 ==
  Bin : Inport
  A : Inport  Port=2
  B : Inport  Port=3
  Logical Operator : Logic  Operator=XOR  IconShape=distinctive  AllPortsSameDT=off  OutDataTypeStr=boolean
  Logical Operator1 : Logic  IconShape=distinctive  AllPortsSameDT=off  OutDataTypeStr=boolean
  Logical Operator2 : Logic  Operator=NOT  IconShape=distinctive  AllPortsSameDT=off  OutDataTypeStr=boolean
  Logical Operator3 : Logic  Operator=OR  IconShape=distinctive  AllPortsSameDT=off  OutDataTypeStr=boolean
  Logical Operator4 : Logic  Operator=XOR  IconShape=distinctive  AllPortsSameDT=off  OutDataTypeStr=boolean
  Logical Operator5 : Logic  IconShape=distinctive  AllPortsSameDT=off  OutDataTypeStr=boolean
  Logical Operator6 : Logic  Operator=NOT  IconShape=distinctive  AllPortsSameDT=off  OutDataTypeStr=boolean
  Diff : Outport
  Bout : Outport  Port=2
  wires:
  Logical Operator4/1 -> Diff/1
  Logical Operator3/1 -> Bout/1
  Logical Operator5/1 -> Logical Operator3/1
  Logical Operator1/1 -> Logical Operator3/2
  A/1 -> Logical Operator/1, Logical Operator2/1
  B/1 -> Logical Operator/2, Logical Operator1/2
  Logical Operator6/1 -> Logical Operator5/1
  Bin/1 -> Logical Operator5/2, Logical Operator4/1
  Logical Operator2/1 -> Logical Operator1/1
  Logical Operator/1 -> Logical Operator4/2, Logical Operator6/1

== system cpusimuilater/ALU/subtractor/sub2 ==
  A : Inport
  B : Inport  Port=2
  Bin : Inport  Port=3
  Logical Operator : Logic  Operator=XOR  IconShape=distinctive  AllPortsSameDT=off  OutDataTypeStr=boolean
  Logical Operator1 : Logic  IconShape=distinctive  AllPortsSameDT=off  OutDataTypeStr=boolean
  Logical Operator2 : Logic  Operator=NOT  IconShape=distinctive  AllPortsSameDT=off  OutDataTypeStr=boolean
  Logical Operator3 : Logic  Operator=OR  IconShape=distinctive  AllPortsSameDT=off  OutDataTypeStr=boolean
  Logical Operator4 : Logic  Operator=XOR  IconShape=distinctive  AllPortsSameDT=off  OutDataTypeStr=boolean
  Logical Operator5 : Logic  IconShape=distinctive  AllPortsSameDT=off  OutDataTypeStr=boolean
  Logical Operator6 : Logic  Operator=NOT  IconShape=distinctive  AllPortsSameDT=off  OutDataTypeStr=boolean
  Diff : Outport
  Bout : Outport  Port=2
  wires:
  Logical Operator4/1 -> Diff/1
  Logical Operator3/1 -> Bout/1
  Logical Operator5/1 -> Logical Operator3/1
  Logical Operator1/1 -> Logical Operator3/2
  A/1 -> Logical Operator/1, Logical Operator2/1
  B/1 -> Logical Operator/2, Logical Operator1/2
  Logical Operator6/1 -> Logical Operator5/1
  Bin/1 -> Logical Operator5/2, Logical Operator4/1
  Logical Operator2/1 -> Logical Operator1/1
  Logical Operator/1 -> Logical Operator4/2, Logical Operator6/1

== system cpusimuilater/ALU/subtractor/sub3 ==
  A : Inport
  B : Inport  Port=2
  Bin : Inport  Port=3
  Logical Operator : Logic  Operator=XOR  IconShape=distinctive  AllPortsSameDT=off  OutDataTypeStr=boolean
  Logical Operator1 : Logic  IconShape=distinctive  AllPortsSameDT=off  OutDataTypeStr=boolean
  Logical Operator2 : Logic  Operator=NOT  IconShape=distinctive  AllPortsSameDT=off  OutDataTypeStr=boolean
  Logical Operator3 : Logic  Operator=OR  IconShape=distinctive  AllPortsSameDT=off  OutDataTypeStr=boolean
  Logical Operator4 : Logic  Operator=XOR  IconShape=distinctive  AllPortsSameDT=off  OutDataTypeStr=boolean
  Logical Operator5 : Logic  IconShape=distinctive  AllPortsSameDT=off  OutDataTypeStr=boolean
  Logical Operator6 : Logic  Operator=NOT  IconShape=distinctive  AllPortsSameDT=off  OutDataTypeStr=boolean
  Diff : Outport
  Bout : Outport  Port=2
  wires:
  Logical Operator4/1 -> Diff/1
  Logical Operator3/1 -> Bout/1
  Logical Operator5/1 -> Logical Operator3/1
  Logical Operator1/1 -> Logical Operator3/2
  A/1 -> Logical Operator/1, Logical Operator2/1
  B/1 -> Logical Operator/2, Logical Operator1/2
  Logical Operator6/1 -> Logical Operator5/1
  Bin/1 -> Logical Operator5/2, Logical Operator4/1
  Logical Operator2/1 -> Logical Operator1/1
  Logical Operator/1 -> Logical Operator4/2, Logical Operator6/1

== system cpusimuilater/ALU/subtractor/sub4 ==
  A : Inport
  B : Inport  Port=2
  Bin : Inport  Port=3
  Logical Operator : Logic  Operator=XOR  IconShape=distinctive  AllPortsSameDT=off  OutDataTypeStr=boolean
  Logical Operator1 : Logic  IconShape=distinctive  AllPortsSameDT=off  OutDataTypeStr=boolean
  Logical Operator2 : Logic  Operator=NOT  IconShape=distinctive  AllPortsSameDT=off  OutDataTypeStr=boolean
  Logical Operator3 : Logic  Operator=OR  IconShape=distinctive  AllPortsSameDT=off  OutDataTypeStr=boolean
  Logical Operator4 : Logic  Operator=XOR  IconShape=distinctive  AllPortsSameDT=off  OutDataTypeStr=boolean
  Logical Operator5 : Logic  IconShape=distinctive  AllPortsSameDT=off  OutDataTypeStr=boolean
  Logical Operator6 : Logic  Operator=NOT  IconShape=distinctive  AllPortsSameDT=off  OutDataTypeStr=boolean
  Diff : Outport
  Bout : Outport  Port=2
  wires:
  Logical Operator4/1 -> Diff/1
  Logical Operator3/1 -> Bout/1
  Logical Operator5/1 -> Logical Operator3/1
  Logical Operator1/1 -> Logical Operator3/2
  A/1 -> Logical Operator/1, Logical Operator2/1
  B/1 -> Logical Operator/2, Logical Operator1/2
  Logical Operator6/1 -> Logical Operator5/1
  Bin/1 -> Logical Operator5/2, Logical Operator4/1
  Logical Operator2/1 -> Logical Operator1/1
  Logical Operator/1 -> Logical Operator4/2, Logical Operator6/1

== system cpusimuilater/ProgramCounter/Adder1/Subsystem ==
  A : Inport
  B : Inport  Port=2
  C : Inport  Port=3
  Logical Operator : Logic  Operator=XOR  IconShape=distinctive  AllPortsSameDT=off  OutDataTypeStr=boolean
  Logical Operator1 : Logic  IconShape=distinctive  AllPortsSameDT=off  OutDataTypeStr=boolean
  Logical Operator2 : Logic  Operator=NOT  IconShape=distinctive  AllPortsSameDT=off  OutDataTypeStr=boolean
  Logical Operator3 : Logic  Operator=OR  IconShape=distinctive  AllPortsSameDT=off  OutDataTypeStr=boolean
  Logical Operator4 : Logic  Operator=XOR  IconShape=distinctive  AllPortsSameDT=off  OutDataTypeStr=boolean
  Logical Operator5 : Logic  IconShape=distinctive  AllPortsSameDT=off  OutDataTypeStr=boolean
  Logical Operator6 : Logic  Operator=NOT  IconShape=distinctive  AllPortsSameDT=off  OutDataTypeStr=boolean
  Sum : Outport
  CarryOut : Outport  Port=2
  wires:
  Logical Operator/1 -> Logical Operator6/1, Logical Operator4/2
  Logical Operator5/1 -> Logical Operator3/1
  Logical Operator1/1 -> Logical Operator3/2
  Logical Operator4/1 -> Sum/1
  Logical Operator2/1 -> Logical Operator1/1
  Logical Operator3/1 -> CarryOut/1
  A/1 -> Logical Operator2/1, Logical Operator/1
  C/1 -> Logical Operator4/1, Logical Operator5/2
  Logical Operator6/1 -> Logical Operator5/1
  B/1 -> Logical Operator1/2, Logical Operator/2

== system cpusimuilater/ProgramCounter/Adder1/Subsystem1 ==
  A : Inport
  B : Inport  Port=2
  C : Inport  Port=3
  Logical Operator : Logic  Operator=XOR  IconShape=distinctive  AllPortsSameDT=off  OutDataTypeStr=boolean
  Logical Operator1 : Logic  IconShape=distinctive  AllPortsSameDT=off  OutDataTypeStr=boolean
  Logical Operator2 : Logic  Operator=NOT  IconShape=distinctive  AllPortsSameDT=off  OutDataTypeStr=boolean
  Logical Operator3 : Logic  Operator=OR  IconShape=distinctive  AllPortsSameDT=off  OutDataTypeStr=boolean
  Logical Operator4 : Logic  Operator=XOR  IconShape=distinctive  AllPortsSameDT=off  OutDataTypeStr=boolean
  Logical Operator5 : Logic  IconShape=distinctive  AllPortsSameDT=off  OutDataTypeStr=boolean
  Logical Operator6 : Logic  Operator=NOT  IconShape=distinctive  AllPortsSameDT=off  OutDataTypeStr=boolean
  Sum : Outport
  CarryOut : Outport  Port=2
  wires:
  Logical Operator/1 -> Logical Operator6/1, Logical Operator4/2
  Logical Operator5/1 -> Logical Operator3/1
  Logical Operator1/1 -> Logical Operator3/2
  Logical Operator4/1 -> Sum/1
  Logical Operator2/1 -> Logical Operator1/1
  Logical Operator3/1 -> CarryOut/1
  A/1 -> Logical Operator2/1, Logical Operator/1
  C/1 -> Logical Operator4/1, Logical Operator5/2
  Logical Operator6/1 -> Logical Operator5/1
  B/1 -> Logical Operator1/2, Logical Operator/2

== system cpusimuilater/ProgramCounter/Adder1/Subsystem2 ==
  A : Inport
  B : Inport  Port=2
  C : Inport  Port=3
  Logical Operator : Logic  Operator=XOR  IconShape=distinctive  AllPortsSameDT=off  OutDataTypeStr=boolean
  Logical Operator1 : Logic  IconShape=distinctive  AllPortsSameDT=off  OutDataTypeStr=boolean
  Logical Operator2 : Logic  Operator=NOT  IconShape=distinctive  AllPortsSameDT=off  OutDataTypeStr=boolean
  Logical Operator3 : Logic  Operator=OR  IconShape=distinctive  AllPortsSameDT=off  OutDataTypeStr=boolean
  Logical Operator4 : Logic  Operator=XOR  IconShape=distinctive  AllPortsSameDT=off  OutDataTypeStr=boolean
  Logical Operator5 : Logic  IconShape=distinctive  AllPortsSameDT=off  OutDataTypeStr=boolean
  Logical Operator6 : Logic  Operator=NOT  IconShape=distinctive  AllPortsSameDT=off  OutDataTypeStr=boolean
  Sum : Outport
  CarryOut : Outport  Port=2
  wires:
  Logical Operator/1 -> Logical Operator6/1, Logical Operator4/2
  Logical Operator5/1 -> Logical Operator3/1
  Logical Operator1/1 -> Logical Operator3/2
  Logical Operator4/1 -> Sum/1
  Logical Operator2/1 -> Logical Operator1/1
  Logical Operator3/1 -> CarryOut/1
  A/1 -> Logical Operator2/1, Logical Operator/1
  C/1 -> Logical Operator4/1, Logical Operator5/2
  Logical Operator6/1 -> Logical Operator5/1
  B/1 -> Logical Operator1/2, Logical Operator/2

== system cpusimuilater/ProgramCounter/Adder1/Subsystem3 ==
  A : Inport
  B : Inport  Port=2
  C : Inport  Port=3
  Logical Operator : Logic  Operator=XOR  IconShape=distinctive  AllPortsSameDT=off  OutDataTypeStr=boolean
  Logical Operator1 : Logic  IconShape=distinctive  AllPortsSameDT=off  OutDataTypeStr=boolean
  Logical Operator2 : Logic  Operator=NOT  IconShape=distinctive  AllPortsSameDT=off  OutDataTypeStr=boolean
  Logical Operator3 : Logic  Operator=OR  IconShape=distinctive  AllPortsSameDT=off  OutDataTypeStr=boolean
  Logical Operator4 : Logic  Operator=XOR  IconShape=distinctive  AllPortsSameDT=off  OutDataTypeStr=boolean
  Logical Operator5 : Logic  IconShape=distinctive  AllPortsSameDT=off  OutDataTypeStr=boolean
  Logical Operator6 : Logic  Operator=NOT  IconShape=distinctive  AllPortsSameDT=off  OutDataTypeStr=boolean
  Sum : Outport
  CarryOut : Outport  Port=2
  wires:
  Logical Operator/1 -> Logical Operator6/1, Logical Operator4/2
  Logical Operator5/1 -> Logical Operator3/1
  Logical Operator1/1 -> Logical Operator3/2
  Logical Operator4/1 -> Sum/1
  Logical Operator2/1 -> Logical Operator1/1
  Logical Operator3/1 -> CarryOut/1
  A/1 -> Logical Operator2/1, Logical Operator/1
  C/1 -> Logical Operator4/1, Logical Operator5/2
  Logical Operator6/1 -> Logical Operator5/1
  B/1 -> Logical Operator1/2, Logical Operator/2

== stateflow chart cpusimuilater/stateMac ==
  state start
    PCenable=0;InstrRegEn=0;DecoderEnable=0;ALUenable=0;RegisterWriteEnable=0;
  state Fetch
    PCenable=1;InstrRegEn=1;DecoderEnable=0;ALUenable=0;RegisterWriteEnable=0;
  state Decode
    PCenable=0;InstrRegEn=0;DecoderEnable=1;ALUenable=0;RegisterWriteEnable=0;
  state Execute
    PCenable=0;InstrRegEn=0;DecoderEnable=0;ALUenable=1;RegisterWriteEnable=0;
  state Writeback
    PCenable=0;InstrRegEn=0;DecoderEnable=0;ALUenable=0;RegisterWriteEnable=1;
  (default) -> start
  start -> Fetch
  Writeback -> Fetch : [delay>40]
  Fetch -> Decode : [delay>10]
  Decode -> Execute : [delay>20]
  Execute -> Writeback : [delay>30]
  data: delay input; PCenable output; InstrRegEn output; DecoderEnable output; ALUenable output; RegisterWriteEnable output
